simulink model "modelo"  (R2018b)
settings: Solver=VariableStepAuto  StartTime=0.0  StopTime=240000  RelTol=1e-3
undefined symbols (not defined in the file or in its folder): f
libraries: instrumentlib x2, fuzblock x1, commrandsrc3 x1
settings Model: Creator=root  LastModifiedBy=root
settings SFSimCC: SimUseLocalCustomCode=off
settings RTWCC: RTWUseLocalCustomCode=off

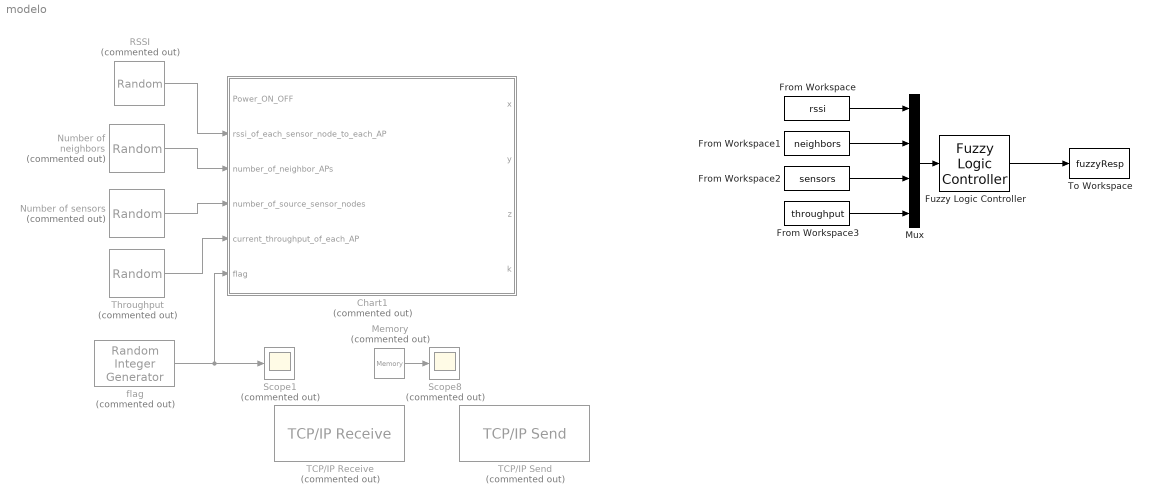
== system modelo ==
  Chart1 : Stateflow chart  Commented=on  TreatAsAtomicUnit=on
  From Workspace : FromWorkspace  VariableName=rssi  SampleTime=0  OutputAfterFinalValue=Cyclic repetition
  From Workspace1 : FromWorkspace  VariableName=neighbors  SampleTime=0  OutputAfterFinalValue=Cyclic repetition
  From Workspace2 : FromWorkspace  VariableName=sensors  SampleTime=0  OutputAfterFinalValue=Cyclic repetition
  From Workspace3 : FromWorkspace  VariableName=throughput  SampleTime=0  OutputAfterFinalValue=Cyclic repetition
  Fuzzy Logic Controller : fuzblock/Fuzzy Logic  Controller  FIS=originalFuzzy  OutputSampleNumber=101  DataType=double  FuzzifiedInputs=off  RuleFiringStrengths=off  RuleOutputs=off  AggregatedOutputs=off  SimulateUsing=Interpreted execution  OutOfRangeInputValueMessage=warning  NoRuleFiredMessage=warning  EmptyOutputFuzzySetMessage=warning
  Memory : Memory  Commented=on
  Mux : Mux
  Number of neighbors : UniformRandomNumber  Commented=on  Minimum=0  Maximum=8  SampleTime=1000
  Number of sensors : UniformRandomNumber  Commented=on  Minimum=0  Maximum=254  Seed=0  SampleTime=1000
  RSSI : UniformRandomNumber  Commented=on  Minimum=-80  Maximum=-40  SampleTime=1000
  Scope1 : Scope  Commented=on
  Scope8 : Scope  Commented=on
  TCP/IP Receive : instrumentlib/TCP//IP Receive  Commented=on  Host=localhost  Port=18638  DataSize=[1 1]  EnableBlockingMode=on  Timeout=10  SampleTime=0.01  DataType=uint8  ByteOrder=BigEndian  ASCIIFormatting=%f,  Terminator=LF
      settings: SourceProductName=Instrument Control Toolbox
  TCP/IP Send : instrumentlib/TCP//IP Send  Commented=on  Port=80  EnableBlockingMode=on  Timeout=10  ByteOrder=BigEndian  TransferDelay=on
      settings: SourceProductName=Instrument Control Toolbox
  Throughput : UniformRandomNumber  Commented=on  Minimum=0  Maximum=100  SampleTime=1000
  To Workspace : ToWorkspace  VariableName=fuzzyResp  SampleTime=-1
      settings: Save2DSignal=2-D array (concatenate along first dimension)
  "flag " : commrandsrc3/Random Integer Generator  Commented=on  SetSize=2  SeedSource=Auto  Seed=0  SampleTime=1000  SamplesPerFrame=1  OutputDataType=single  SimulateUsing=Interpreted execution
      settings: SourceProductName=Communications Toolbox
  wires:
  Mux/1 -> Fuzzy Logic Controller/1
  Memory/1 -> Scope8/1
  "flag "/1 -> Chart1/6(flag), Scope1/1
  Number of sensors/1 -> Chart1/4(number_of_source_sensor_nodes)
  Throughput/1 -> Chart1/5(current_throughput_of_each_AP)
  RSSI/1 -> Chart1/2(rssi_of_each_sensor_node_to_each_AP)
  Number of neighbors/1 -> Chart1/3(number_of_neighbor_APs)
  From Workspace/1 -> Mux/1
  From Workspace1/1 -> Mux/2
  From Workspace3/1 -> Mux/4
  From Workspace2/1 -> Mux/3
  Fuzzy Logic Controller/1 -> To Workspace/1

== stateflow chart modelo/Chart1 ==
  state ActiveState
    entry:  x = rssi_of_each_sensor_node_to_each_AP;
    y = number_of_neighbor_APs;
    z = number_of_source_sensor_nodes;
    k = current_throughput_of_each_AP;
    Power_ON_OFF<50%
  state SleepState
    entry: Power_ON_OFF>50%;
  state Start
  SleepState -> ActiveState [order 1] : [flag == 1]
  ActiveState -> ActiveState [order 2] : [flag == 1]
  (default) -> Start
  SleepState -> SleepState [order 2] : [flag == 0]
  Start -> ActiveState [order 2] : [flag == 1]
  Start -> SleepState [order 1] : [flag == 0]
  ActiveState -> SleepState [order 1] : [flag == 0]
  data: Power_ON_OFF input; rssi_of_each_sensor_node_to_each_AP input; number_of_neighbor_APs input; number_of_source_sensor_nodes input; current_throughput_of_each_AP input; x output; y output; z output; k output; flag input
